simulink model "Problem_4"  (R2020a)
settings: Solver=VariableStepAuto  StartTime=0.0  StopTime=10.0  RelTol=1e-3
settings Model: Creator=user  LastModifiedBy=user

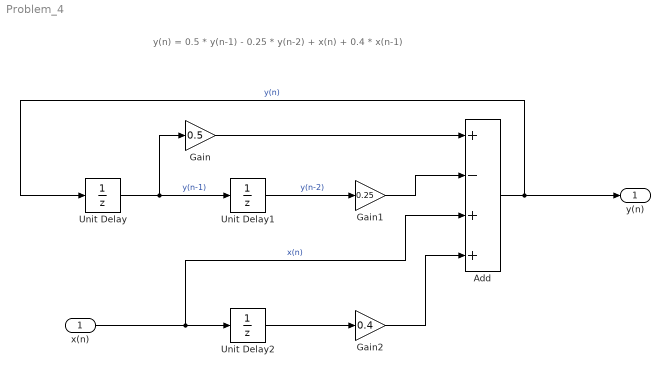
== system Problem_4 ==
  note: y(n) = 0.5 * y(n-1) - 0.25 * y(n-2) + x(n) + 0.4 * x(n-1)
  x(n) : Inport
  Add : Sum  Inputs=+-++
  Gain : Gain  Gain=0.5
  Gain1 : Gain  Gain=0.25
  Gain2 : Gain  Gain=0.4
  Unit Delay : UnitDelay  SampleTime=-1  HasFrameUpgradeWarning=on
  Unit Delay1 : UnitDelay  SampleTime=-1  HasFrameUpgradeWarning=on
  Unit Delay2 : UnitDelay  SampleTime=-1  HasFrameUpgradeWarning=on
  y(n) : Outport
  wires:
  Unit Delay/1 -> Gain/1, Unit Delay1/1  "y(n-1)"
  Unit Delay1/1 -> Gain1/1  "y(n-2)"
  Gain/1 -> Add/1
  Gain1/1 -> Add/2
  Unit Delay2/1 -> Gain2/1
  Gain2/1 -> Add/4
  x(n)/1 -> Add/3, Unit Delay2/1  "x(n)"
  Add/1 -> y(n)/1, Unit Delay/1  "y(n)"
